simulink model "CarLQR_Sim"  (R2019a)
settings: Solver=VariableStepAuto  StartTime=0.0  StopTime=20  RelTol=1e-3
values from neighbouring files (symbols this model uses):
  A = [-rho*Area*Cv*v0/m]    [CarLQR.m]    (also in SpeedControlWithIntegral.m)
  Area = 2.4    [CarLQR.m]    (also in SpeedControlWithIntegral.m)
  B = [1/m]    [CarLQR.m]    (also in SpeedControlWithIntegral.m)
  C = [1]    [CarLQR.m]    (also in SpeedControlWithIntegral.m)
  Cr = 0.01    [CarLQR.m]    (also in SpeedControlWithIntegral.m)
  Cv = 0.32    [CarLQR.m]    (also in SpeedControlWithIntegral.m)
  D = 0    [CarLQR.m]    (also in SpeedControlWithIntegral.m)
  delay = 0.2    [CarLQR.m]    (also in SpeedControlWithIntegral.m)
  F = Fe(1)    [CarLQR.m]    (also in SpeedControlWithIntegral.m)
  g = 9.81    [CarLQR.m]    (also in SpeedControlWithIntegral.m)
  H = Fe(2)    [CarLQR.m]    (also in SpeedControlWithIntegral.m)
  m = 1400    [CarLQR.m]    (also in SpeedControlWithIntegral.m = 2037)
  rho = 1.3    [CarLQR.m]    (also in SpeedControlWithIntegral.m)
  tauAct = 0.1    [CarLQR.m]    (also in SpeedControlWithIntegral.m)
  u0 = 0.5*rho*Area*Cv*v0^2 + m*g*Cr    (= 378.9528)    [CarLQR.m]    (also in SpeedControlWithIntegral.m = 441.4425)
  v0 = 22    [CarLQR.m]    (also in SpeedControlWithIntegral.m)
libraries: simulink x2
settings Model: Creator=DELL  LastModifiedBy=DELL

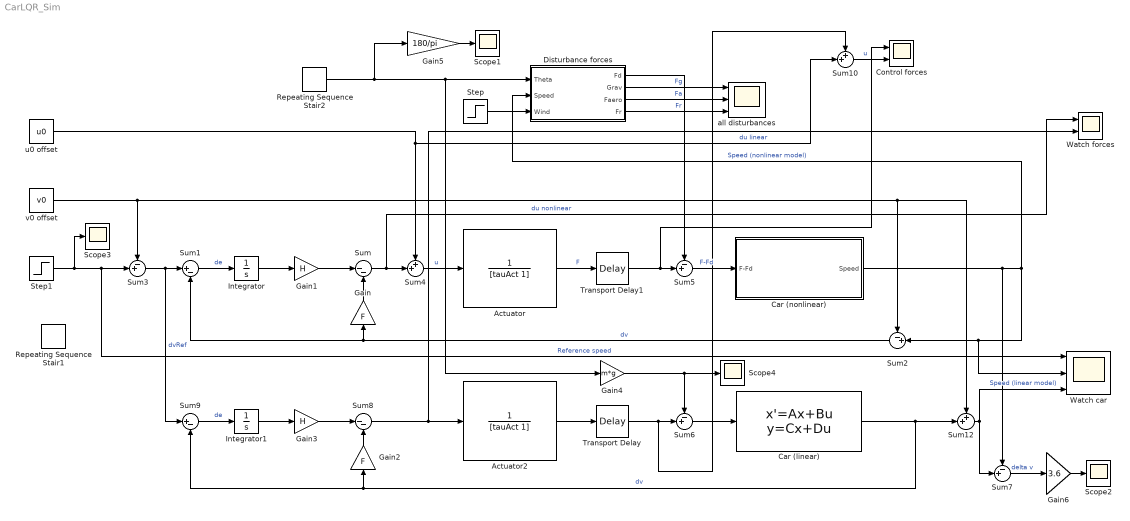
== system CarLQR_Sim ==
  Actuator : TransferFcn  Denominator=[tauAct 1]
  Actuator2 : TransferFcn  Denominator=[tauAct 1]
  Car (linear) : StateSpace  A=A  B=B  C=C  D=D  InitialCondition=-5
  Car (nonlinear) : Subsystem
  Control forces : Scope  NumInputPorts=2
  Disturbance forces : Subsystem
  Gain : Gain  Gain=F
  Gain1 : Gain  Gain=H
  Gain2 : Gain  Gain=F
  Gain3 : Gain  Gain=H
  Gain4 : Gain  Gain=m*g
  Gain5 : Gain  Gain=180/pi
  Gain6 : Gain  Gain=3.6
  Integrator : Integrator
  Integrator1 : Integrator
  Repeating Sequence Stair1 : simulink/Sources/Repeating Sequence Stair  OutValues=[25 30].'  tsamp=200  OutMin=[]  OutMax=[]  OutDataTypeStr=double  OutputDataTypeScalingMode=double  OutDataType=fixdt(0,8)  ConRadixGroup=Best Precision: Vector-wise  OutScaling=2^-12
  Repeating Sequence Stair2 : simulink/Sources/Repeating Sequence Stair  OutValues=0*[0 0.02 0.05 0.01].'  tsamp=10  OutMin=[]  OutMax=[]  OutDataTypeStr=double  OutputDataTypeScalingMode=double  OutDataType=fixdt(0,8)  ConRadixGroup=Best Precision: Vector-wise  OutScaling=2^-12
  Scope{1..4} (4 alike) : Scope
  Step : Step  Time=20  After=0*120/3.6  SampleTime=0
  Step1 : Step  Time=0  After=25  SampleTime=0
  Sum : Sum  Inputs=|--
  Sum1 : Sum  Inputs=|+-
  Sum10 : Sum  Inputs=++|
  Sum12 : Sum  Inputs=++|
  Sum{2..3,5..7} (5 alike) : Sum  Inputs=-+|
  Sum4 : Sum  Inputs=++|
  Sum8 : Sum  Inputs=|--
  Sum9 : Sum  Inputs=|+-
  Transport Delay : TransportDelay  DelayTime=delay
  Transport Delay1 : TransportDelay  DelayTime=delay
  Watch car : Scope  NumInputPorts=3
  Watch forces : Scope  NumInputPorts=2
  all disturbances : Scope  NumInputPorts=3
  u0 offset : Constant  Value=u0
  "v0 offset " : Constant  Value=v0
  wires:
  Gain5/1 -> Scope1/1
  Disturbance forces/1(Fd) -> Sum5/1
  Gain6/1 -> Scope2/1
  Step/1 -> Disturbance forces/3(Wind)
  Sum10/1 -> Control forces/2  "u"
  Sum2/1 -> Sum1/2, Gain/1  "dv"
  Disturbance forces/4(Fr) -> all disturbances/3  "Fr"
  Sum5/1 -> Car (nonlinear)/1("F-Fd ")  "F-Fd"
  Gain/1 -> Sum/2
  Car (nonlinear)/1(Speed) -> Sum7/1, Watch car/2, Sum2/2, Disturbance forces/2(Speed)  "Speed (nonlinear model)"
  Sum12/1 -> Watch car/3, Sum7/2  "Speed (linear model)"
  Actuator/1 -> Transport Delay1/1  "F"
  Gain2/1 -> Sum8/2
  Sum4/1 -> Actuator/1  "u"
  Step1/1 -> Scope3/1, Watch car/1, Sum3/2  "Reference speed"
  Integrator/1 -> Gain1/1
  "v0 offset "/1 -> Sum12/1, Sum2/1, Sum3/1
  Car (linear)/1 -> Sum12/2, Sum9/2, Gain2/1  "dv"
  Disturbance forces/2(Grav) -> all disturbances/1  "Fg"
  Gain3/1 -> Sum8/1
  Sum7/1 -> Gain6/1  "delta v"
  Integrator1/1 -> Gain3/1
  Gain4/1 -> Scope4/1, Sum6/1
  u0 offset/1 -> Sum10/2, Sum4/1
  Sum6/1 -> Car (linear)/1
  Sum3/1 -> Sum9/1, Sum1/1  "dvRef"
  Gain1/1 -> Sum/1
  Disturbance forces/3(Faero) -> all disturbances/2  "Fa"
  Actuator2/1 -> Transport Delay/1
  Sum/1 -> Watch forces/1, Sum4/2  "du nonlinear"
  Sum9/1 -> Integrator1/1  "de"
  Sum8/1 -> Watch forces/2, Actuator2/1  "du linear"
  Sum1/1 -> Integrator/1  "de"
  Transport Delay/1 -> Sum10/1, Sum6/2
  Transport Delay1/1 -> Control forces/1, Sum5/2
  Repeating Sequence Stair2/1 -> Gain5/1, Gain4/1, Disturbance forces/1(Theta)

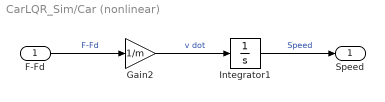
== system CarLQR_Sim/Car (nonlinear) ==
  "F-Fd " : Inport
  Gain2 : Gain  Gain=1/m
  Integrator1 : Integrator  InitialCondition=20
  Speed : Outport
  wires:
  Gain2/1 -> Integrator1/1  "v dot"
  "F-Fd "/1 -> Gain2/1  "F-Fd"
  Integrator1/1 -> Speed/1  "Speed"

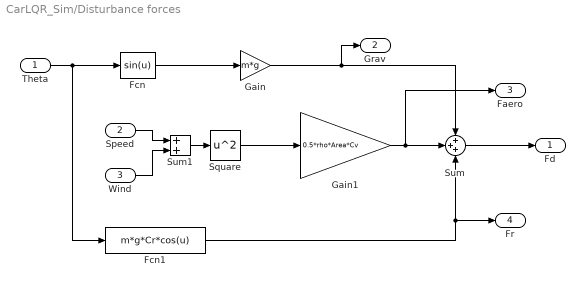
== system CarLQR_Sim/Disturbance forces ==
  Theta : Inport
  Speed : Inport  Port=2
  Wind : Inport  Port=3
  Fcn : Fcn  Expr=sin(u)
  Fcn1 : Fcn  Expr=m*g*Cr*cos(u)
  Gain : Gain  Gain=m*g
  Gain1 : Gain  Gain=0.5*rho*Area*Cv
  Square : Math  Operator=square  SaturateOnIntegerOverflow=on
  Sum : Sum  Inputs=+++
  Sum1 : Sum
  Fd : Outport
  Grav : Outport  Port=2
  Faero : Outport  Port=3
  Fr : Outport  Port=4
  wires:
  Theta/1 -> Fcn1/1, Fcn/1
  Square/1 -> Gain1/1
  Gain/1 -> Grav/1, Sum/1
  Gain1/1 -> Faero/1, Sum/2
  Fcn1/1 -> Fr/1, Sum/3
  Sum/1 -> Fd/1
  Fcn/1 -> Gain/1
  Sum1/1 -> Square/1
  Speed/1 -> Sum1/1
  Wind/1 -> Sum1/2
